simulink model "t"  (R2020b)
settings: Solver=VariableStepAuto  StartTime=0.0  StopTime=10.0  RelTol=1e-3
values from neighbouring files (symbols this model uses):
  b = 0.05    [t.m]
  k = 0.1    [t.m]
  m = 500    [t.m]
undefined symbols (not defined in the file or in its folder): g
settings Model: Creator=HP  LastModifiedBy=HP

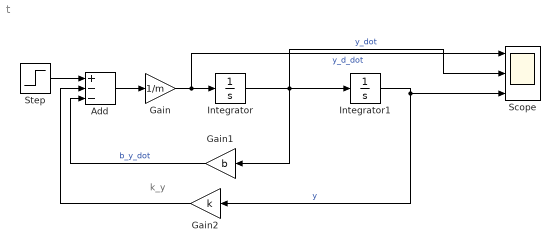
== system t ==
  note: k_y
  Add : Sum  Inputs=+--
  Gain : Gain  Gain=1/m
  Gain1 : Gain  Gain=b
  Gain2 : Gain  Gain=k
  Integrator : Integrator  InitialCondition=10
  Integrator1 : Integrator
  Scope : Scope  NumInputPorts=3
  Step : Step  After=g  SampleTime=0
  wires:
  Gain/1 -> Scope/1, Integrator/1  "y_d_dot"
  Add/1 -> Gain/1
  Integrator1/1 -> Scope/3, Gain2/1  "y"
  Integrator/1 -> Scope/2, Gain1/1, Integrator1/1  "y_dot"
  Gain2/1 -> Add/2
  Step/1 -> Add/1
  Gain1/1 -> Add/3  "b_y_dot"
